simulink model "cv_small_controller"  (Simulink 6.0)
settings: Solver=ode45  StartTime=0.0  StopTime=10.0  RelTol=1e-3
settings Model: RecordCoverage=on  CovMetricSettings=dcmtrw  Creator=The MathWorks Inc.  LastModifiedBy=batserve  ExtModeAutoUpdateStatusClock=off  ProdHWDeviceType=Specified
settings DataIOCC: SignalLoggingName=logsOut
settings OptimizationCC: BlockReduction=off  ConditionallyExecuteInputs=off
settings DebuggingCC: CheckExecutionContextPreStartOutputMsg=on  CheckExecutionContextRuntimeOutputMsg=on  SolverPrmCheckMsg=none
settings HardwareCC: ProdHWDeviceType=Specified

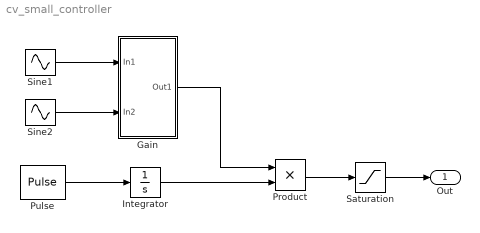
== system cv_small_controller ==
  Gain : Subsystem  PropExecContextAcrossSSBoundary=on
  Integrator : Integrator
  Product : Product  RndMeth=Zero
  Pulse : DiscretePulseGenerator  PulseType=Time based  PulseWidth=50
  Saturation : Saturate
  Sine1 : Sin  Amplitude=3  Bias=5.5  SampleTime=0
  Sine2 : Sin  Amplitude=3  Bias=5.5  Phase=pi/2  SampleTime=0
  Out : Outport
  wires:
  Product/1 -> Saturation/1
  Gain/1(Out1) -> Product/1
  Saturation/1 -> Out/1
  Pulse/1 -> Integrator/1
  Integrator/1 -> Product/2
  Sine1/1 -> Gain/1(In1)
  Sine2/1 -> Gain/2(In2)

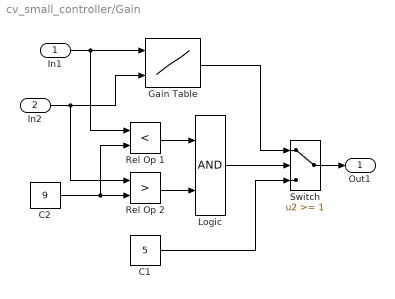
== system cv_small_controller/Gain ==
  In1 : Inport  Port=1  LatchInput=off
  In2 : Inport  Port=2  LatchInput=off
  C1 : Constant  Value=5
  C2 : Constant  Value=9
  Gain Table : Lookup2D  DialogController=Simulink.DDGSource  RowIndex=[1:10]  ColumnIndex=[1:10]  OutputValues=sqrt([1:10]'*[1:10])
  Logic : Logic  AllPortsSameDT=off  OutDataTypeMode=Boolean
  Rel Op 1 : RelationalOperator  Operator=<  LogicOutDataTypeMode=Boolean
  Rel Op 2 : RelationalOperator  Operator=>  LogicOutDataTypeMode=Boolean
  Switch : Switch  Threshold=1
  Out1 : Outport
  wires:
  C1/1 -> Switch/3
  Gain Table/1 -> Switch/1
  In1/1 -> Rel Op 1/1, Gain Table/1
  In2/1 -> Rel Op 2/1, Gain Table/2
  Logic/1 -> Switch/2
  C2/1 -> Rel Op 2/2, Rel Op 1/2
  Rel Op 1/1 -> Logic/1
  Rel Op 2/1 -> Logic/2
  Switch/1 -> Out1/1
